simulink model "es_2_2"  (R2024b)
settings: Solver=VariableStepAuto  StartTime=0.0  StopTime=30  RelTol=1e-3
undefined symbols (not defined in the file or in its folder): dspblkCoreblockFVToolHelper, gcbh
libraries: vrlib x1
settings Model: Creator=mattia  LastModifiedBy=elima

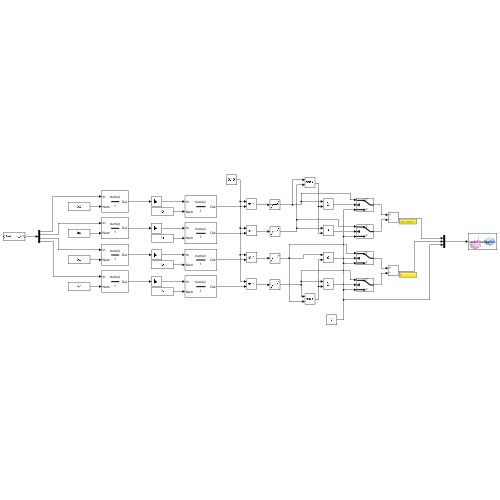
[thumbnail: Simulink's stored preview of the top-level diagram]
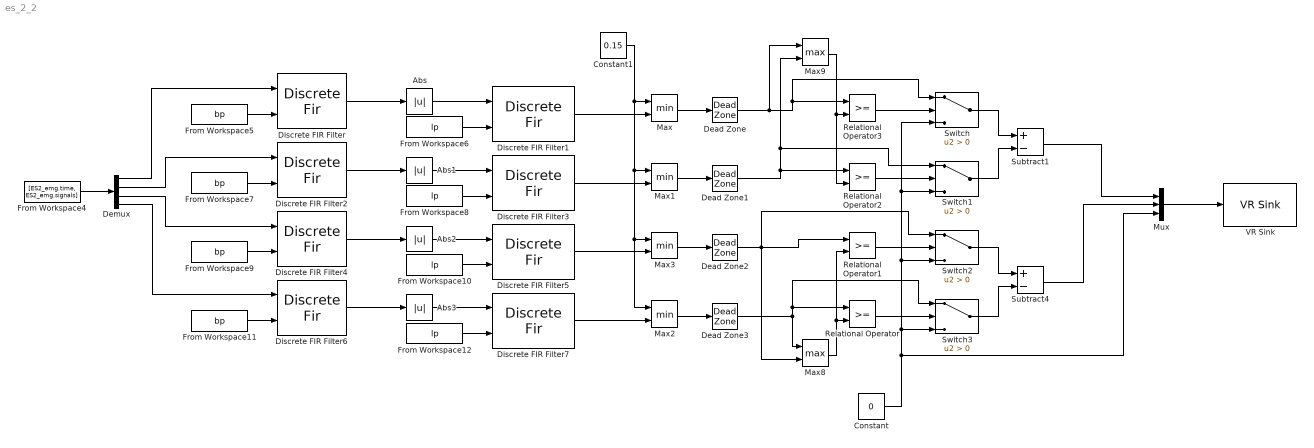
== system es_2_2 ==
  Abs{,1..3} (4 alike) : Abs  SaturateOnIntegerOverflow=off
  Constant : Constant  Value=0  OutDataTypeStr=double
  Constant1 : Constant  Value=0.15
  Dead Zone{,1..3} (4 alike) : DeadZone  LowerValue=-0.05  UpperValue=0.05
  Demux : Demux
  Discrete FIR Filter{,1..7} (8 alike) : DiscreteFir  LoadFcn=dspblkCoreblockFVToolHelper(gcbh,'load');  CoefSource=Input port
      settings: CopyFcn=dspblkCoreblockFVToolHelper(gcbh,'copy');  DeleteFcn=dspblkCoreblockFVToolHelper(gcbh,'close');  ModelCloseFcn=dspblkCoreblockFVToolHelper(gcbh,'close');  PreSaveFcn=dspblkCoreblockFVToolHelper(gcbh,'presave');  PostSaveFcn=dspblkCoreblockFVToolHelper(gcbh,'postsave');  CloseFcn=dspblkCoreblockFVToolHelper(gcbh,'close');  InputPortMap=u0,u1
  From Workspace{6,8,10,12} (4 alike) : FromWorkspace  VariableName=lp
  From Workspace{5,7,9,11} (4 alike) : FromWorkspace  VariableName=bp
  From Workspace4 : FromWorkspace  VariableName=[ES2_emg.time, ES2_emg.signals]  SampleTime=-1
  Max{,1..3} (4 alike) : MinMax  Inputs=2
  Max8 : MinMax  Function=max  Inputs=2
  Max9 : MinMax  Function=max  Inputs=2
  Mux : Mux  Inputs=3
  Relational Operator{,1..3} (4 alike) : RelationalOperator  OutDataTypeStr=boolean  RndMeth=Simplest  InputSameDT=off
  Subtract1 : Sum  Inputs=+-  OutDataTypeStr=double
  Subtract4 : Sum  Inputs=+-  OutDataTypeStr=double
  Switch{,1..3} (4 alike) : Switch  Criteria=u2 > Threshold  SaturateOnIntegerOverflow=off  InputSameDT=off
  VR Sink : vrlib/VR Sink  InstantiateOnLoad=on  SampleTime=0.1  ViewEnable=on  RemoteChange=off  RemoteView=off  FieldsWritten=cursor.translation.3.1.1.double  WorldFileName=8_palline_color.wrl  AutoView=off  VideoDimensions=[]  AllowVariableSize=off
  wires:
  Mux/1 -> VR Sink/1
  From Workspace4/1 -> Demux/1
  Discrete FIR Filter/1 -> Abs/1
  Abs/1 -> Discrete FIR Filter1/1
  From Workspace5/1 -> Discrete FIR Filter/2
  From Workspace6/1 -> Discrete FIR Filter1/2
  Discrete FIR Filter2/1 -> Abs1/1
  Abs1/1 -> Discrete FIR Filter3/1
  From Workspace8/1 -> Discrete FIR Filter3/2
  From Workspace7/1 -> Discrete FIR Filter2/2
  Discrete FIR Filter4/1 -> Abs2/1
  Abs2/1 -> Discrete FIR Filter5/1
  From Workspace10/1 -> Discrete FIR Filter5/2
  From Workspace9/1 -> Discrete FIR Filter4/2
  Discrete FIR Filter6/1 -> Abs3/1
  Abs3/1 -> Discrete FIR Filter7/1
  From Workspace12/1 -> Discrete FIR Filter7/2
  From Workspace11/1 -> Discrete FIR Filter6/2
  Demux/1 -> Discrete FIR Filter/1
  Demux/2 -> Discrete FIR Filter2/1
  Demux/3 -> Discrete FIR Filter4/1
  Demux/4 -> Discrete FIR Filter6/1
  Constant1/1 -> Max2/1, Max3/1, Max1/1, Max/1
  Relational Operator2/1 -> Switch1/2
  Relational Operator3/1 -> Switch/2
  Relational Operator1/1 -> Switch2/2
  Relational Operator/1 -> Switch3/2
  Switch2/1 -> Subtract4/1
  Switch3/1 -> Subtract4/2
  Switch/1 -> Subtract1/1
  Switch1/1 -> Subtract1/2
  Max9/1 -> Relational Operator2/2, Relational Operator3/2
  Max8/1 -> Relational Operator1/2, Relational Operator/2
  Discrete FIR Filter5/1 -> Max3/2
  Discrete FIR Filter7/1 -> Max2/2
  Discrete FIR Filter1/1 -> Max/2
  Discrete FIR Filter3/1 -> Max1/2
  Constant/1 -> Mux/3, Switch/3, Switch1/3, Switch2/3, Switch3/3
  Subtract1/1 -> Mux/1
  Subtract4/1 -> Mux/2
  Max/1 -> Dead Zone/1
  Max1/1 -> Dead Zone1/1
  Max3/1 -> Dead Zone2/1
  Max2/1 -> Dead Zone3/1
  Dead Zone3/1 -> Relational Operator/1, Switch3/1, Max8/1
  Dead Zone2/1 -> Switch2/1, Relational Operator1/1, Max8/2
  Dead Zone1/1 -> Max9/2, Switch1/1, Relational Operator2/1
  Dead Zone/1 -> Max9/1, Switch/1, Relational Operator3/1
